simulink model "test2"  (R2016a)
settings: Solver=FixedStepAuto  SolverMode=SingleTasking  StartTime=0.0  StopTime=inf  FixedStep=5e-6  RelTol=1e-3
PreLoadFcn:
  | waijung.modelPreload; % Required for working with Waijung Blockset. Do not remove.
undefined symbols (not defined in the file): ARM, HSEOSC, Link, LQFP100, MDK, ST, STM32F407VE
libraries: simulink x8, powerlib_meascontrol x1, etargetslib x1, stm32f4_adc_lib x1, stm32f4_device_config_lib x1
CloseFcn:
  | waijung.modelClose; % Required for working with Waijung Blockset. Do not remove.
settings Model: Creator=Dang Khoa  LastModifiedBy=Dang Khoa
settings OptimizationCC: DefaultParameterBehavior=Inlined  OptimizeModelRefInitCode=on  LifeSpan=1
settings HardwareCC: ProdBitPerPointer=32  ProdLargestAtomicInteger=Long  ProdWordSize=32  ProdHWDeviceType=ARM Compatible->ARM 10  TargetEndianess=LittleEndian  TargetHWDeviceType=ARM Compatible->Cortex - M4
settings RTWCC: SystemTargetFile=stm32f4.tlc  GenCodeOnly=on  GenerateMakefile=off  TemplateMakefile=ert_default_tmf  Description=STM32F4 Target  GenerateReport=on  IncludeHyperlinkInReport=on  LaunchReport=on  GenerateTraceInfo=on  GenerateTraceReport=on  GenerateTraceReportSl=on  GenerateTraceReportSf=on  GenerateTraceReportEml=on
settings CodeAppCC: ForceParamTrailComments=on  IgnoreCustomStorageClasses=off  OperatorAnnotations=on  SimulinkDataObjDesc=on  SFDataObjDesc=on  MATLABFcnDesc=on  InsertBlockDesc=on  MATLABSourceComments=on
settings STFCustomTargetCC: ModelReferenceCompliant=off  CombineOutputUpdateFcns=on  ERTCustomFileBanners=on  SupportContinuousTime=off  SupportNonInlinedSFcns=off  MATLABClassNameForMDSCustomization=Simulink.SoftwareTarget.ERTCustomization  GRTInterface=off  SystemTargetFile=stm32f4.tlc
settings ERTTargetCC: ModelReferenceCompliant=off  ParMdlRefBuildCompliant=off  CompOptLevelCompliant=off  ConcurrentExecutionCompliant=off  ERTFirstTimeCompliant=off  ModelStepFunctionPrototypeControlCompliant=off  CPPClassGenCompliant=off  UseToolchainInfoCompliant=off  InlinedParameterPlacement=NonHierarchical  ERTSrcFileBannerTemplate=stm32f4_code_template.cgt  ERTHdrFileBannerTemplate=stm32f4_code_template.cgt  ERTDataSrcFileTemplate=stm32f4_code_template.cgt  ERTDataHdrFileTemplate=stm32f4_code_template.cgt  ERTCustomFileTemplate=stm32f4_file_process.tlc

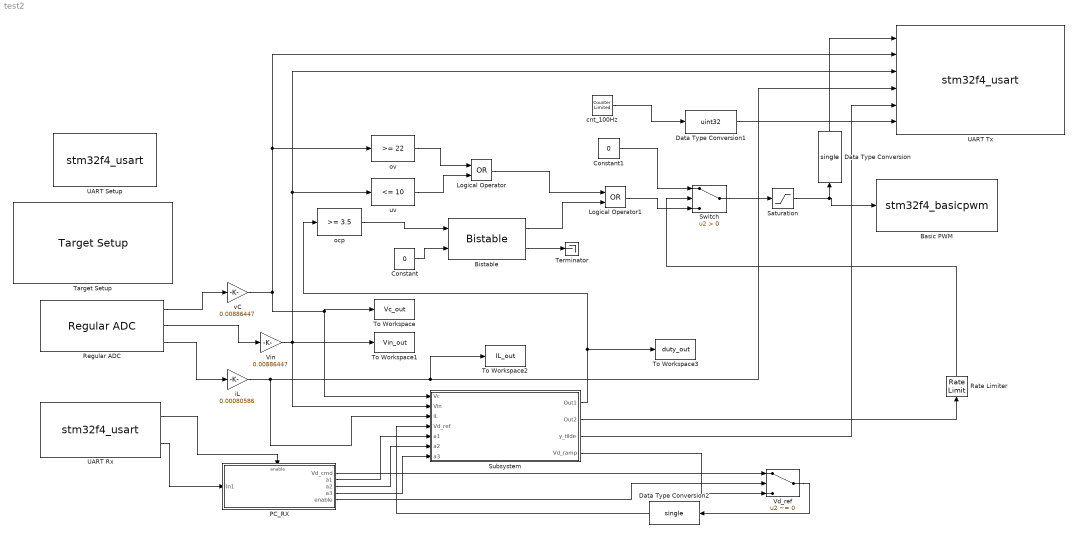
== system test2 ==
  Basic PWM : S-Function  FunctionName=stm32f4_basicpwm  Parameters=timer,pwmperiod,ch1pin,ch2pin,ch3pin,ch4pin,sampletime,sampletimestr,blockid,apb,portstr,pinstr,pinmat,timarr,timprescale,chmat,polaritystr  SFunctionDeploymentMode=off  EnableBusSupport=off  mask(stm32f4_basicpwm){timer=4, pwmperiod=1/20000, polarity=Active High, polaritystr=TIM_OCPolarity_High, ch1pin=B6, ch2pin=Not available - Do not use, ch3pin=Not available - Do not use, ch4pin=Not available - Do not use, sampletime=-1, sampletimestr=5e-05, blockid=BasicPWM, portpinstr=B6,,,, enablecustomportlabel=off, cinputportlabel=In1, In2, In3, In4, coutputportlabel=0, apb=1, portstr=["B"], pinstr=["GPIO_Pin_6"], pinmat=[1 6], timarr=64614, timprescale=25, chmat=[1]}
      mask prompts: pwmperiod "PWM Period (seconds)"; ch1pin "Channel 1"; ch2pin "Channel 2"; ch3pin "Channel 3"; ch4pin "Channel 4"; sampletime "Sample time (sec)"; sampletimestr "Compiled sample time (sec) in string"; portpinstr "Port pin string"; enablecustomportlabel "Enable custom port labels"; cinputportlabel "Custom input port labels (Ex. In1, In2, In3)"; coutputportlabel "Custom output port labels (Ex. Out1, Out2, Out3)"; portstr "Port string"; pinstr "Pin string"; pinmat "Pin matrix"; timarr "Timer ARR"; timprescale "Timer PRESCALE"; chmat "Channel order"
      mask help:
      | This block implements basic Edge-aligned Pulse Width Modulation (PWM) generation.
      | All timers are 16-bit. The PWM period is fixed (per timer).
      mask init:
      | stm32f4_basicpwm_callback('init');
      mask Help: web(fullfile(waijungdocroot,'stm32f4_basicpwm.htm'),'-browser')
      mask TypeOptions timer: 1 | 2 | 3 | 4 | 5 | 8 | 9 | 10 | 11 | 12 | 13 | 14
      mask Callback timer: stm32f4_basicpwm_callback('timer');
      mask Callback pwmperiod: stm32f4_basicpwm_callback('pwmperiod');
      mask TypeOptions polarity: Active High | Active Low
      mask Callback polarity: stm32f4_basicpwm_callback('polarity');
      mask TypeOptions ch1pin: Not available - Do not use | B6 | D12
      mask Callback ch1pin: stm32f4_basicpwm_callback('ch1pin');
      mask TypeOptions ch2pin: Not available - Do not use | B7 | D13
      mask Callback ch2pin: stm32f4_basicpwm_callback('ch2pin');
      mask TypeOptions ch3pin: Not available - Do not use | B8 | D14
      mask Callback ch3pin: stm32f4_basicpwm_callback('ch3pin');
      mask TypeOptions ch4pin: Not available - Do not use | B9 | D15
      mask Callback ch4pin: stm32f4_basicpwm_callback('ch4pin');
      mask Callback sampletime: stm32f4_basicpwm_callback('sampletime');
      mask Callback sampletimestr: stm32f4_basicpwm_callback('sampletimestr');
      mask Callback blockid: stm32f4_basicpwm_callback('blockid');
      mask Callback enablecustomportlabel: stm32f4_basicpwm_callback('enablecustomportlabel');
      mask Display: text(0.95, 0.5, 'Timer: 4\nPolarity: Active High\nPeriod (sec) 1/20000\nTs (sec): 5e-05','ver','middle','hor','right');port_label('input', 1,'CH1 (B6)')
  Bistable : powerlib_meascontrol/Logic/Bistable  Qpriority=Set  ic=0  Ts=-1
  Constant : Constant  Value=0
  Constant1 : Constant  Value=0
  Data Type Conversion : DataTypeConversion  OutDataTypeStr=single
  Data Type Conversion1 : DataTypeConversion  OutDataTypeStr=uint32
  Data Type Conversion2 : DataTypeConversion  OutDataTypeStr=single
  Logical Operator : Logic  Operator=OR  AllPortsSameDT=off  OutDataTypeStr=boolean
  Logical Operator1 : Logic  Operator=OR  AllPortsSameDT=off  OutDataTypeStr=boolean
  PC_RX : Subsystem  TreatAsAtomicUnit=on
  Rate Limiter : RateLimiter  RisingSlewLimit=2000  FallingSlewLimit=-4000  SampleTimeMode=inherited
  Regular ADC : stm32f4_adc_lib/Regular ADC  adcmodule=1  outputdatatype=Single  prescaler=2  prescalerstr=ADC_Prescaler_Div2  chsamplingtime=Auto  chsamplingtimestr=ADC_SampleTime_480Cycles  read_an0=off  read_an1=off  read_an2=off  read_an3=off  read_an4=off  read_an5=off  read_an6=off  read_an7=off  read_an8=off  read_an9=off  read_an10=on  read_an11=on  read_an12=on  read_an13=off  read_an14=off  read_an15=off  read_an16=off  read_an17=off  read_an18=off  pinstr=GPIO_Pin_10 | GPIO_Pin_11 | GPIO_Pin_12  usedpinarray="[0  0  0  0  0  0  0  0  0  0  1  1  1  0  0  0  0  0  0]"  usedportidarray="[2  2  2]"  usedpinidarray="[0  1  2]"  usedpinidcount=3  sampletime=5e-5  blockid=RegularADC  enablecustomportlabel=off  cinputportlabel=0  coutputportlabel=Out1, Out2
  Saturation : Saturate  UpperLimit=1  LowerLimit=0
  Subsystem : Subsystem
  Switch : Switch  Criteria=u2 > Threshold
  Target Setup : stm32f4_device_config_lib/Target Setup  Priority=100  compiler=MDK-ARM  previous_compiler=MDK-ARM  mcu=STM32F407VE (LQFP100)  mcustr=STM32F407VE  clockconfig=HSEOSC-8MHz  system_stm32f4xx_c_path=D:\MATLAB\setup\waijung17_03a\targets\stm32f4_target\stm32f4\utils\system_stm32f4xx_default\STM32F40_41xxx\hseosc8mhz  showmemoryconfiguration=off  stacksize=0x2000  heapsize=0x2000  enableautocompiledownload=on  fullchiperase=off  programmerinterface=ST-Link  editctrlstr=on  compilercontrolstr=-c --cpu Cortex-M4.fp -g -O3 --apcs=interwork --split_sections $(INCLUDES)  assemblercontrolstr="--cpu Cortex-M4.fp -g --apcs=interwork  --xref $(INCLUDES)"  linkercontrolstr="--cpu Cortex-M4.fp --strict --scatter \"$(MODELNAME).sct\" --summary_stderr --info summarysizes --map --xref --callgraph --symbols --info sizes --info totals --info unused --info veneers  --list \".\\$(MODELNAME).map\" -o $(MODELNAME).axf"  runafterdownload=on  execprofile=Real-time output  profileruart=3  profilerbaud=500000  profilertxpin=D8  profilerinitstr=5e-5,168000000,8400,500000,0  manualsetsampletime=on  sampletime=5e-5  blockid=TargetSetup  systickreloadvalue=8400  hseval=8000000  lastprofileruart=3  hclk=168000000  flashorigin=0x08000000  flashlength=0x80000  ramorigin=0x20000000  ramlength=0x20000  useextram=off
  Terminator : Terminator
  To Workspace : ToWorkspace  VariableName=Vc_out  SampleTime=-1
  To Workspace1 : ToWorkspace  VariableName=Vin_out  SampleTime=-1
  To Workspace2 : ToWorkspace  VariableName=IL_out  SampleTime=-1
  To Workspace3 : ToWorkspace  VariableName=duty_out  SampleTime=-1
  UART Rx : S-Function  Priority=1  FunctionName=stm32f4_usart  Parameters=configuration,uartmodule,transfer,baudrate,inputtype,outputtype,confstr,binheaderarray,binterminatorarray,asciiheader,asciiterminator,bindatalength,packetmode,varname,sampletime,sampletimestr,blockid  SFunctionDeploymentMode=off  EnableBusSupport=off  mask(stm32f4_usart){configuration=Rx, uartmodule=2, baudrate=115200, databits=8, parity=No, stopbit=1, remaptxpin=Not used, remaprxpin=Not used, flowcontrol=None, remapctspin=Not used, remaprtspin=Not used, advanceoptions=off, rxbuffersize=512, txbuffersize=512, transfer=Non-Blocking, packetmode=Binary Vector, binheader='00', binterminator='', porttype_double=0, porttype_single=0, porttype_int8=0, porttype_uint8=19, porttype_int16=0, porttype_uint16=0, porttype_int32=0, porttype_uint32=0, asciiformat='value=%d,%f', rx_asciiterminator=CRLF (0x0D 0x0A - "\r\n"), tx_asciiterminator=LF (0x0A - "\n"), storagename=<empty>, varname=, inputtype=[0], outputtype=[2 3  4867], binheaderarray=[1 0], binterminatorarray=[0 ], bindatalength=19, asciiheader='value=%d,%f\r\n', asciiterminator=[2 13 10], sampletime=5e-5, sampletimestr=5e-05, blockid=UARTRx, confstr=[ "dummy", "0", "*", "*", "0", "*", "*", "0", "*", "*", "0", "*", "*", "1", "4", "6", "1", "4", "5", "512", "512", "1", "2", "115200", "8", "No", "1", "None", "USART2"], lastmodule=1}
      mask prompts: uartmodule "UART Module"; baudrate "Baud rate (bps)"; databits "Data bits"; stopbit "Stop bit"; remaptxpin "Tx Pin"; remaprxpin "Rx Pin"; flowcontrol "Hardware flow control"; remapctspin "HW Flow control, CTS Pin"; remaprtspin "HW Flow control, RTS Pin"; advanceoptions "Advance options"; rxbuffersize "Rx buffer size (bytes)"; txbuffersize "Tx buffer size (bytes)"; packetmode "Packet mode"; binheader "Binary header (example: '7E 7E')"; binterminator "Binary terminator (example: '03 03')"; porttype_double "Number of data port, type DOUBLE"; porttype_single "Number of data port, type SINGLE"; porttype_int8 "Number of data port, type INT8"; porttype_uint8 "Number of data port, type UINT8"; porttype_int16 "Number of data port, type INT16"; porttype_uint16 "Number of data port, type UINT16"; porttype_int32 "Number of data port, type INT32"; porttype_uint32 "Number of data port, type UINT32"; asciiformat "Ascii format"; rx_asciiterminator "End of packet"; tx_asciiterminator "End of packet"; storagename "Buffer"; varname "Var name"; inputtype "Input data type"; outputtype "Output data type"; binheaderarray "Binary header"; binterminatorarray "Binary terminator"; bindatalength "Binary data length"; asciiheader "Ascii header (printf format)"; asciiterminator "Ascii terminator"; sampletime "Sample time (sec)"; sampletimestr "Compiled sample time (sec) in string"; confstr "Configuration string"; lastmodule "Last module selected"
      mask help:
      | Data type for Ascii format
      | %u, %i, %d, %o, %x: uint32
      | %e, %g, %f: single
      | %c: int8
      mask init:
      | stm32f4_usart_callback('init');
      mask Help: web(fullfile(waijungdocroot,'stm32f4_usart_rx.htm'), '-browser')
      mask TypeOptions configuration: Setup | Tx | Rx
      mask Callback configuration: stm32f4_usart_callback('configuration');
      mask TypeOptions uartmodule: 1 | 2 | 3 | 4 | 5 | 6
      mask Callback uartmodule: stm32f4_usart_callback('uartmodule');
      mask Callback baudrate: stm32f4_usart_callback('baudrate');
      mask TypeOptions databits: 8
      mask TypeOptions parity: No | Odd | Even
      mask TypeOptions stopbit: 0.5 | 1 | 1.5 | 2
      mask TypeOptions remaptxpin: Not used | A9 | B6
      mask TypeOptions remaprxpin: Not used | A10 | B7
      mask TypeOptions flowcontrol: None | RTS | CTS | RTS/CTS
      mask Callback flowcontrol: stm32f4_usart_callback('flowcontrol');
      mask TypeOptions remapctspin: Not used | A11
      mask TypeOptions remaprtspin: Not used | A12
      mask Callback advanceoptions: stm32f4_usart_callback('advanceoptions');
      mask TypeOptions rxbuffersize: 16 | 32 | 64 | 128 | 256 | 512 | 1024 | 2048
      mask TypeOptions txbuffersize: 16 | 32 | 64 | 128 | 256 | 512 | 1024 | 2048
      mask TypeOptions transfer: Blocking | Non-Blocking
      mask Callback transfer: stm32f4_usart_callback('transfer');
      mask TypeOptions packetmode: Ascii | Binary | Binary Vector | String Buffer | Raw Buffer | Read Line
      mask Callback packetmode: stm32f4_usart_callback('packetmode');
      mask Callback binheader: stm32f4_usart_callback('binheader');
      mask Callback binterminator: stm32f4_usart_callback('binterminator');
      mask Callback porttype_double: stm32f4_usart_callback('porttype');
      mask Callback porttype_single: stm32f4_usart_callback('porttype');
      mask Callback porttype_int8: stm32f4_usart_callback('porttype');
      mask Callback porttype_uint8: stm32f4_usart_callback('porttype');
      mask Callback porttype_int16: stm32f4_usart_callback('porttype');
      mask Callback porttype_uint16: stm32f4_usart_callback('porttype');
      mask Callback porttype_int32: stm32f4_usart_callback('porttype');
      mask Callback porttype_uint32: stm32f4_usart_callback('porttype');
      mask Callback asciiformat: stm32f4_usart_callback('asciiformat');
      mask TypeOptions rx_asciiterminator: CR (0x0D - "\r") | LF (0x0A - "\n") | CRLF (0x0D 0x0A - "\r\n")
      mask Callback rx_asciiterminator: stm32f4_usart_callback('rx_asciiterminator');
      mask TypeOptions tx_asciiterminator: CR (0x0D - "\r") | LF (0x0A - "\n") | CRLF (0x0D 0x0A - "\r\n") | None
      mask Callback tx_asciiterminator: stm32f4_usart_callback('tx_asciiterminator');
      mask TypeOptions storagename: <empty>
      mask Callback storagename: stm32f4_usart_callback('storagename');
      mask Callback varname: stm32f4_usart_callback('varname');
      mask Callback sampletime: stm32f4_usart_callback('sampletime');
      mask Callback sampletimestr: stm32f4_usart_callback('sampletimestr');
      mask Callback blockid: stm32f4_usart_callback('blockid');
      mask Display: text(0.05, 0.5, 'Module: USART2_Rx\nPacket: Binary Vector\nTransfer: Non-Blocking\nTs (sec): 5e-05','ver','middle','hor','left'); port_label('output', 1,'READY'); port_label('output', 2,'uint8(19)');
  UART Setup : S-Function  Priority=1  FunctionName=stm32f4_usart  Parameters=configuration,uartmodule,transfer,baudrate,inputtype,outputtype,confstr,binheaderarray,binterminatorarray,asciiheader,asciiterminator,bindatalength,packetmode,varname,sampletime,sampletimestr,blockid  SFunctionDeploymentMode=off  EnableBusSupport=off  mask(stm32f4_usart){configuration=Setup, uartmodule=2, baudrate=115200, databits=8, parity=No, stopbit=1, remaptxpin=A2, remaprxpin=A3, flowcontrol=None, remapctspin=Not used, remaprtspin=Not used, advanceoptions=off, rxbuffersize=512, txbuffersize=512, transfer=Blocking, packetmode=Ascii, binheader='7E 7E', binterminator='03 03', porttype_double=1, porttype_single=0, porttype_int8=1, porttype_uint8=0, porttype_int16=0, porttype_uint16=0, porttype_int32=0, porttype_uint32=0, asciiformat='%d,%f', rx_asciiterminator=CRLF (0x0D 0x0A - "\r\n"), tx_asciiterminator=CR (0x0D - "\r"), storagename=<empty>, varname=, inputtype=[0], outputtype=[0], binheaderarray=[0], binterminatorarray=[0], bindatalength=0, asciiheader='', asciiterminator=[0], sampletime=-1, sampletimestr=5e-05, blockid=UARTSetup, confstr=[ "dummy", "1", "A", "2", "1", "A", "3", "0", "*", "*", "0", "*", "*", "1", "4", "6", "1", "4", "5", "512", "512", "1", "2", "115200", "8", "No", "1", "None", "USART2"], lastmodule=2}
      mask prompts: uartmodule "UART Module"; baudrate "Baud rate (bps)"; databits "Data bits"; stopbit "Stop bit"; remaptxpin "Tx Pin"; remaprxpin "Rx Pin"; flowcontrol "Hardware flow control"; remapctspin "HW Flow control, CTS Pin"; remaprtspin "HW Flow control, RTS Pin"; advanceoptions "Advance options"; rxbuffersize "Rx buffer size (bytes)"; txbuffersize "Tx buffer size (bytes)"; packetmode "Packet mode"; binheader "Binary header (example: '7E 7E')"; binterminator "Binary terminator (example: '03 03')"; porttype_double "Number of data port, type DOUBLE"; porttype_single "Number of data port, type SINGLE"; porttype_int8 "Number of data port, type INT8"; porttype_uint8 "Number of data port, type UINT8"; porttype_int16 "Number of data port, type INT16"; porttype_uint16 "Number of data port, type UINT16"; porttype_int32 "Number of data port, type INT32"; porttype_uint32 "Number of data port, type UINT32"; asciiformat "Ascii format"; rx_asciiterminator "End of packet"; tx_asciiterminator "End of packet"; storagename "Buffer"; varname "Var name"; inputtype "Input data type"; outputtype "Output data type"; binheaderarray "Binary header"; binterminatorarray "Binary terminator"; bindatalength "Binary data length"; asciiheader "Ascii header (printf format)"; asciiterminator "Ascii terminator"; sampletime "Sample time (sec)"; sampletimestr "Compiled sample time (sec) in string"; confstr "Configuration string"; lastmodule "Last module selected"
      mask help:
      | Default STM32F4DISCOVERY + aMG F4 Connect 2 + aMG USB Converter N2 settings use
      |
      | USART3, Tx D8, Rx D9 and USB Serial Converter A.
      mask init:
      | stm32f4_usart_callback('init');
      mask Help: web(fullfile(waijungdocroot,'stm32f4_usart_setup.htm'), '-browser')
      mask TypeOptions configuration: Setup | Tx | Rx
      mask Callback configuration: stm32f4_usart_callback('configuration');
      mask TypeOptions uartmodule: 1 | 2 | 3 | 4 | 5 | 6
      mask Callback uartmodule: stm32f4_usart_callback('uartmodule');
      mask Callback baudrate: stm32f4_usart_callback('baudrate');
      mask TypeOptions databits: 8
      mask TypeOptions parity: No | Odd | Even
      mask TypeOptions stopbit: 0.5 | 1 | 1.5 | 2
      mask TypeOptions remaptxpin: Not used | A2 | D5
      mask TypeOptions remaprxpin: Not used | A3 | D6
      mask TypeOptions flowcontrol: None | RTS | CTS | RTS/CTS
      mask Callback flowcontrol: stm32f4_usart_callback('flowcontrol');
      mask TypeOptions remapctspin: Not used | A0 | D3
      mask TypeOptions remaprtspin: Not used | A1 | D4
      mask Callback advanceoptions: stm32f4_usart_callback('advanceoptions');
      mask TypeOptions rxbuffersize: 16 | 32 | 64 | 128 | 256 | 512 | 1024 | 2048
      mask TypeOptions txbuffersize: 16 | 32 | 64 | 128 | 256 | 512 | 1024 | 2048
      mask TypeOptions transfer: Blocking | Non-Blocking
      mask Callback transfer: stm32f4_usart_callback('transfer');
      mask TypeOptions packetmode: Ascii | Binary | String Buffer
      mask Callback packetmode: stm32f4_usart_callback('packetmode');
      mask Callback binheader: stm32f4_usart_callback('binheader');
      mask Callback binterminator: stm32f4_usart_callback('binterminator');
      mask Callback porttype_double: stm32f4_usart_callback('porttype');
      mask Callback porttype_single: stm32f4_usart_callback('porttype');
      mask Callback porttype_int8: stm32f4_usart_callback('porttype');
      mask Callback porttype_uint8: stm32f4_usart_callback('porttype');
      mask Callback porttype_int16: stm32f4_usart_callback('porttype');
      mask Callback porttype_uint16: stm32f4_usart_callback('porttype');
      mask Callback porttype_int32: stm32f4_usart_callback('porttype');
      mask Callback porttype_uint32: stm32f4_usart_callback('porttype');
      mask Callback asciiformat: stm32f4_usart_callback('asciiformat');
      mask TypeOptions rx_asciiterminator: CR (0x0D - "\r") | LF (0x0A - "\n") | CRLF (0x0D 0x0A - "\r\n")
      mask Callback rx_asciiterminator: stm32f4_usart_callback('rx_asciiterminator');
      mask TypeOptions tx_asciiterminator: CR (0x0D - "\r") | LF (0x0A - "\n") | CRLF (0x0D 0x0A - "\r\n") | None
      mask Callback tx_asciiterminator: stm32f4_usart_callback('tx_asciiterminator');
      mask TypeOptions storagename: <empty>
      mask Callback storagename: stm32f4_usart_callback('storagename');
      mask Callback varname: stm32f4_usart_callback('varname');
      mask Callback sampletime: stm32f4_usart_callback('sampletime');
      mask Callback sampletimestr: stm32f4_usart_callback('sampletimestr');
      mask Callback blockid: stm32f4_usart_callback('blockid');
      mask Display: text(0.5, 0.5, 'Module: USART2_Setup\nBaud (Bps): 115200\nDMA Buffer: 512/512\nTx/Rx Pin: A2/A3','ver','middle','hor','center');
  UART Tx : S-Function  Priority=1  FunctionName=stm32f4_usart  Parameters=configuration,uartmodule,transfer,baudrate,inputtype,outputtype,confstr,binheaderarray,binterminatorarray,asciiheader,asciiterminator,bindatalength,packetmode,varname,sampletime,sampletimestr,blockid  SFunctionDeploymentMode=off  EnableBusSupport=off  mask(stm32f4_usart){configuration=Tx, uartmodule=2, baudrate=115200, databits=8, parity=No, stopbit=1, remaptxpin=Not used, remaprxpin=Not used, flowcontrol=None, remapctspin=Not used, remaprtspin=Not used, advanceoptions=off, rxbuffersize=512, txbuffersize=512, transfer=Non-Blocking, packetmode=Binary, binheader='AA 55', binterminator='', porttype_double=0, porttype_single=5, porttype_int8=0, porttype_uint8=0, porttype_int16=0, porttype_uint16=0, porttype_int32=0, porttype_uint32=1, asciiformat='value=%d,%f', rx_asciiterminator=CRLF (0x0D 0x0A - "\r\n"), tx_asciiterminator=CRLF (0x0D 0x0A - "\r\n"), storagename=<empty>, varname=, inputtype=[6  1 1 1 1 1 7], outputtype=[0], binheaderarray=[2 170   85], binterminatorarray=[0 ], bindatalength=24, asciiheader='value=%d,%f\r\n', asciiterminator=[2 13 10], sampletime=-1, sampletimestr=5e-05, blockid=UARTTx, confstr=[ "dummy", "0", "*", "*", "0", "*", "*", "0", "*", "*", "0", "*", "*", "1", "4", "6", "1", "4", "5", "512", "512", "1", "2", "115200", "8", "No", "1", "None", "USART2"], lastmodule=1}
      mask prompts: uartmodule "UART Module"; baudrate "Baud rate (bps)"; databits "Data bits"; stopbit "Stop bit"; remaptxpin "Tx Pin"; remaprxpin "Rx Pin"; flowcontrol "Hardware flow control"; remapctspin "HW Flow control, CTS Pin"; remaprtspin "HW Flow control, RTS Pin"; advanceoptions "Advance options"; rxbuffersize "Rx buffer size (bytes)"; txbuffersize "Tx buffer size (bytes)"; packetmode "Packet mode"; binheader "Binary header (example: '7E 7E')"; binterminator "Binary terminator (example: '03 03')"; porttype_double "Number of data port, type DOUBLE"; porttype_single "Number of data port, type SINGLE"; porttype_int8 "Number of data port, type INT8"; porttype_uint8 "Number of data port, type UINT8"; porttype_int16 "Number of data port, type INT16"; porttype_uint16 "Number of data port, type UINT16"; porttype_int32 "Number of data port, type INT32"; porttype_uint32 "Number of data port, type UINT32"; asciiformat "Ascii format"; rx_asciiterminator "End of packet"; tx_asciiterminator "End of packet"; storagename "Buffer"; varname "Var name"; inputtype "Input data type"; outputtype "Output data type"; binheaderarray "Binary header"; binterminatorarray "Binary terminator"; bindatalength "Binary data length"; asciiheader "Ascii header (printf format)"; asciiterminator "Ascii terminator"; sampletime "Sample time (sec)"; sampletimestr "Compiled sample time (sec) in string"; confstr "Configuration string"; lastmodule "Last module selected"
      mask help:
      | Data type for Ascii format
      | %u, %i, %d, %o, %x: uint32
      | %e, %g, %f: single
      | %c: int8
      mask init:
      | stm32f4_usart_callback('init');
      mask Help: web(fullfile(waijungdocroot,'stm32f4_usart_tx.htm'), '-browser')
      mask TypeOptions configuration: Setup | Tx | Rx
      mask Callback configuration: stm32f4_usart_callback('configuration');
      mask TypeOptions uartmodule: 1 | 2 | 3 | 4 | 5 | 6
      mask Callback uartmodule: stm32f4_usart_callback('uartmodule');
      mask Callback baudrate: stm32f4_usart_callback('baudrate');
      mask TypeOptions databits: 8
      mask TypeOptions parity: No | Odd | Even
      mask TypeOptions stopbit: 0.5 | 1 | 1.5 | 2
      mask TypeOptions remaptxpin: Not used | A9 | B6
      mask TypeOptions remaprxpin: Not used | A10 | B7
      mask TypeOptions flowcontrol: None | RTS | CTS | RTS/CTS
      mask Callback flowcontrol: stm32f4_usart_callback('flowcontrol');
      mask TypeOptions remapctspin: Not used | A11
      mask TypeOptions remaprtspin: Not used | A12
      mask Callback advanceoptions: stm32f4_usart_callback('advanceoptions');
      mask TypeOptions rxbuffersize: 16 | 32 | 64 | 128 | 256 | 512 | 1024 | 2048
      mask TypeOptions txbuffersize: 16 | 32 | 64 | 128 | 256 | 512 | 1024 | 2048
      mask TypeOptions transfer: Blocking | Non-Blocking
      mask Callback transfer: stm32f4_usart_callback('transfer');
      mask TypeOptions packetmode: Ascii | Binary | Binary Vector | String Buffer | Raw Buffer
      mask Callback packetmode: stm32f4_usart_callback('packetmode');
      mask Callback binheader: stm32f4_usart_callback('binheader');
      mask Callback binterminator: stm32f4_usart_callback('binterminator');
      mask Callback porttype_double: stm32f4_usart_callback('porttype');
      mask Callback porttype_single: stm32f4_usart_callback('porttype');
      mask Callback porttype_int8: stm32f4_usart_callback('porttype');
      mask Callback porttype_uint8: stm32f4_usart_callback('porttype');
      mask Callback porttype_int16: stm32f4_usart_callback('porttype');
      mask Callback porttype_uint16: stm32f4_usart_callback('porttype');
      mask Callback porttype_int32: stm32f4_usart_callback('porttype');
      mask Callback porttype_uint32: stm32f4_usart_callback('porttype');
      mask Callback asciiformat: stm32f4_usart_callback('asciiformat');
      mask TypeOptions rx_asciiterminator: CR (0x0D - "\r") | LF (0x0A - "\n") | CRLF (0x0D 0x0A - "\r\n")
      mask Callback rx_asciiterminator: stm32f4_usart_callback('rx_asciiterminator');
      mask TypeOptions tx_asciiterminator: CR (0x0D - "\r") | LF (0x0A - "\n") | CRLF (0x0D 0x0A - "\r\n") | None
      mask Callback tx_asciiterminator: stm32f4_usart_callback('tx_asciiterminator');
      mask TypeOptions storagename: <empty>
      mask Callback storagename: stm32f4_usart_callback('storagename');
      mask Callback varname: stm32f4_usart_callback('varname');
      mask Callback sampletime: stm32f4_usart_callback('sampletime');
      mask Callback sampletimestr: stm32f4_usart_callback('sampletimestr');
      mask Callback blockid: stm32f4_usart_callback('blockid');
      mask Display: text(0.5, 0.5, 'Module: USART2_Tx\nPacket: Binary\nTransfer: Non-Blocking\nTs (sec): 5e-05','ver','middle','hor','center'); port_label('input', 1,'single'); port_label('input', 2,'single'); port_label('input', 3,'single'); port_label('input', 4,'single'); port_label('input', 5,'single'); port_label('input', 6,'uint32');
  Vd_ref : Switch  Criteria=u2 ~= 0
  Vin : Gain  Gain=0.00886447
  cnt_100Hz : simulink/Sources/Counter Limited  uplimit=199  tsamp=5e-5
  iL : Gain  Gain=0.00080586
  ocp : simulink/Logic and Bit Operations/Compare To Constant  relop=>=  const=3.5  OutDataTypeStr=boolean
  ov : simulink/Logic and Bit Operations/Compare To Constant  relop=>=  const=22  OutDataTypeStr=boolean
  uv : simulink/Logic and Bit Operations/Compare To Constant  relop=<=  const=10  OutDataTypeStr=boolean
  vC : Gain  Gain=0.00886447
  wires:
  Regular ADC/2 -> Vin/1
  Regular ADC/1 -> vC/1
  vC/1 -> UART Tx/2, ov/1, Subsystem/1(Vc), To Workspace/1
  Vin/1 -> To Workspace1/1, UART Tx/3, uv/1, Subsystem/2(Vin)
  uv/1 -> Logical Operator/2
  ov/1 -> Logical Operator/1
  ocp/1 -> Bistable/1
  Constant/1 -> Bistable/2
  Logical Operator/1 -> Logical Operator1/1
  Bistable/1 -> Logical Operator1/2
  Constant1/1 -> Switch/1
  Logical Operator1/1 -> Switch/3
  Rate Limiter/1 -> Switch/2
  Switch/1 -> Saturation/1
  Saturation/1 -> Basic PWM/1, Data Type Conversion/1
  Subsystem/1(Out1) -> To Workspace3/1, ocp/1
  Subsystem/2(Out2) -> Rate Limiter/1
  iL/1 -> To Workspace2/1, UART Tx/4, Subsystem/3("iL ")
  Regular ADC/3 -> iL/1
  Subsystem/3(y_tilde) -> UART Tx/5
  UART Rx/1 -> PC_RX/Enable
  PC_RX/1(Vd_cmd) -> Vd_ref/1
  PC_RX/5(enable) -> Vd_ref/2
  Subsystem/4(Vd_ramp) -> Vd_ref/3
  PC_RX/2(a1) -> Subsystem/5(a1)
  PC_RX/3(a2) -> Subsystem/6(a2)
  PC_RX/4(a3) -> Subsystem/7(a3)
  Bistable/2 -> Terminator/1
  UART Rx/2 -> PC_RX/1(In1)
  Data Type Conversion/1 -> UART Tx/1
  Data Type Conversion1/1 -> UART Tx/6
  cnt_100Hz/1 -> Data Type Conversion1/1
  Vd_ref/1 -> Data Type Conversion2/1
  Data Type Conversion2/1 -> Subsystem/4(Vd_ref)

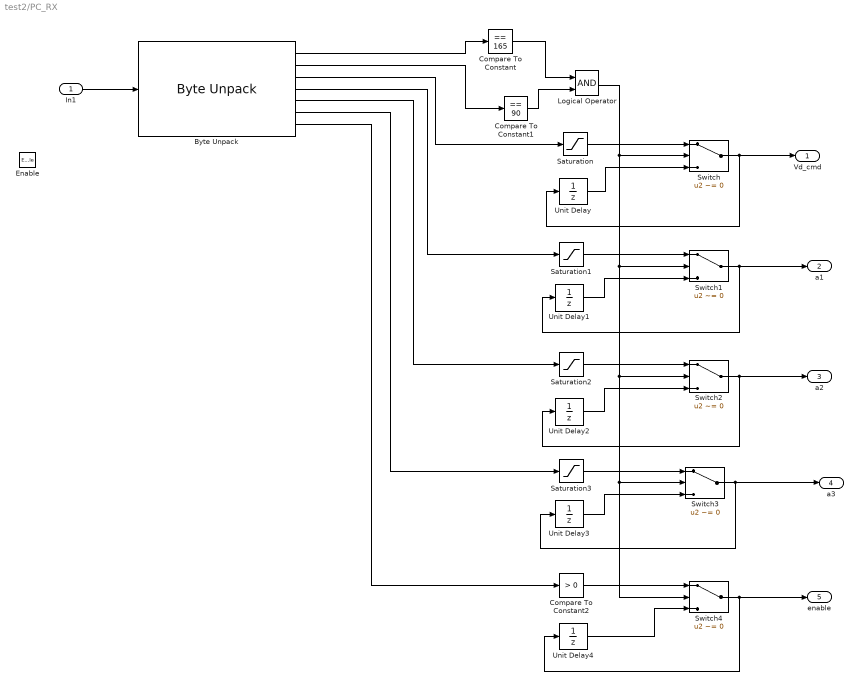
== system test2/PC_RX ==
  In1 : Inport  OutDataTypeStr=uint8  PortDimensions=19
  Enable : EnablePort
  Byte Unpack : etargetslib/Byte Unpack  dimensions={[1],[1],[1],[1],[1],[1],[1]}  datatypes={'uint8','uint8','single','single','single','single','uint8'}  byteAlign=1
  Compare To Constant : simulink/Logic and Bit Operations/Compare To Constant  relop===  const=165  OutDataTypeStr=boolean
  Compare To Constant1 : simulink/Logic and Bit Operations/Compare To Constant  relop===  const=90  OutDataTypeStr=boolean
  Compare To Constant2 : simulink/Logic and Bit Operations/Compare To Constant  relop=>  const=0  OutDataTypeStr=boolean
  Logical Operator : Logic  AllPortsSameDT=off  OutDataTypeStr=boolean
  Saturation : Saturate  UpperLimit=25  LowerLimit=15
  Saturation1 : Saturate  UpperLimit=1  LowerLimit=0
  Saturation2 : Saturate  UpperLimit=0.2  LowerLimit=0
  Saturation3 : Saturate  UpperLimit=0.1  LowerLimit=0
  Switch{,1..4} (5 alike) : Switch  Criteria=u2 ~= 0
  Unit Delay : UnitDelay  InitialCondition=20  SampleTime=-1
  Unit Delay1 : UnitDelay  InitialCondition=0.2  SampleTime=-1
  Unit Delay2 : UnitDelay  SampleTime=-1
  Unit Delay3 : UnitDelay  SampleTime=-1
  Unit Delay4 : UnitDelay  SampleTime=-1
  Vd_cmd : Outport  OutDataTypeStr=single
  a1 : Outport  Port=2  OutDataTypeStr=single
  a2 : Outport  Port=3  OutDataTypeStr=single
  a3 : Outport  Port=4  OutDataTypeStr=single
  enable : Outport  Port=5  OutDataTypeStr=boolean
  wires:
  In1/1 -> Byte Unpack/1
  Compare To Constant/1 -> Logical Operator/1
  Compare To Constant1/1 -> Logical Operator/2
  Byte Unpack/1 -> Compare To Constant/1
  Byte Unpack/2 -> Compare To Constant1/1
  Byte Unpack/3 -> Saturation/1
  Byte Unpack/4 -> Saturation1/1
  Byte Unpack/5 -> Saturation2/1
  Byte Unpack/6 -> Saturation3/1
  Byte Unpack/7 -> Compare To Constant2/1
  Logical Operator/1 -> Switch4/2, Switch3/2, Switch2/2, Switch1/2, Switch/2
  Saturation/1 -> Switch/1
  Saturation1/1 -> Switch1/1
  Saturation2/1 -> Switch2/1
  Saturation3/1 -> Switch3/1
  Compare To Constant2/1 -> Switch4/1
  Unit Delay/1 -> Switch/3
  Switch/1 -> Vd_cmd/1, Unit Delay/1
  Unit Delay1/1 -> Switch1/3
  Switch1/1 -> a1/1, Unit Delay1/1
  Unit Delay2/1 -> Switch2/3
  Switch2/1 -> a2/1, Unit Delay2/1
  Unit Delay3/1 -> Switch3/3
  Switch3/1 -> Unit Delay3/1, a3/1
  Unit Delay4/1 -> Switch4/3
  Switch4/1 -> enable/1, Unit Delay4/1

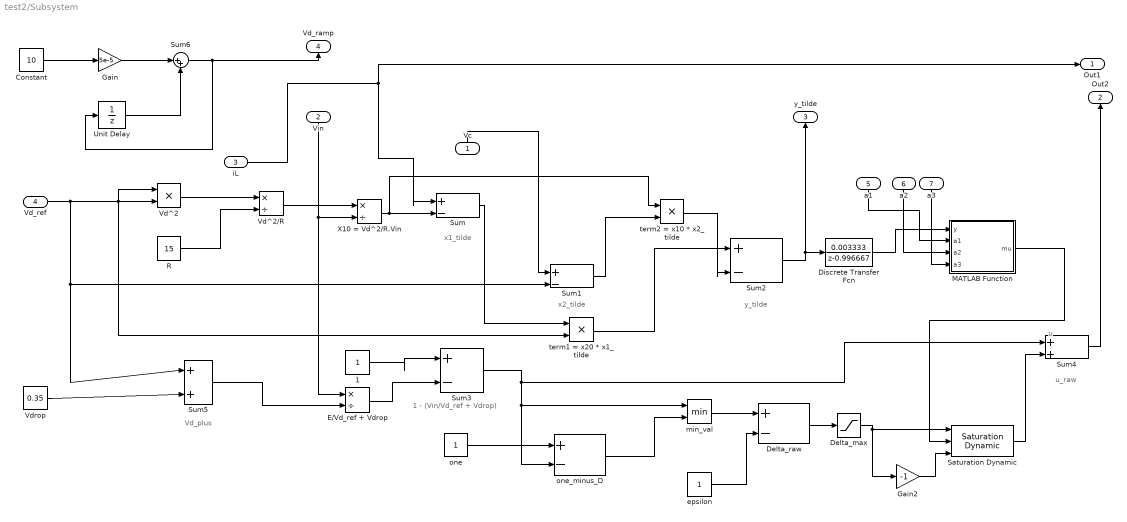
== system test2/Subsystem ==
  note: Vd_plus
  note: u_raw
  note: u
  note: 1 - (Vin/Vd_ref + Vdrop)
  note: x1_tilde
  note: x2_tilde
  note: y_tilde
  Vc : Inport
  Vin : Inport  Port=2
  "iL " : Inport  Port=3
  Vd_ref : Inport  Port=4
  a1 : Inport  Port=5
  a2 : Inport  Port=6
  a3 : Inport  Port=7
  "1 " : Constant
  Constant : Constant  Value=10
  Delta_max : Saturate  UpperLimit=inf  LowerLimit=0
  Delta_raw : Sum  Inputs=+-
  Discrete Transfer Fcn : DiscreteTransferFcn  Numerator=[0.003333]  Denominator=[1 -0.996667]  SampleTime=5e-5
  E/Vd_ref + Vdrop : Product  Inputs=*/
  Gain : Gain  Gain=5e-5
  Gain2 : Gain  Gain=-1  OutDataTypeStr=single
  MATLAB Function : MATLAB Function  TreatAsAtomicUnit=on
  R : Constant  Value=15  OutDataTypeStr=single
  Saturation Dynamic : simulink/Discontinuities/Saturation Dynamic  OutMin=[]  OutMax=[]  OutDataTypeStr=Inherit: Same as second input  OutDataType=fixdt(1, 16)  OutScaling=2^-10  DoSatur=off
  Sum : Sum  Inputs=|+-
  Sum1 : Sum  Inputs=|+-  OutDataTypeStr=Inherit: Same as first input
  Sum2 : Sum  Inputs=|+-
  Sum3 : Sum  Inputs=|+-
  Sum4 : Sum  Inputs=|++
  Sum5 : Sum  Inputs=|++
  Sum6 : Sum  Inputs=|++
  Unit Delay : UnitDelay  SampleTime=5e-5
  Vd^2 : Product  OutDataTypeStr=Inherit: Same as first input
  Vd^2/R : Product  Inputs=*/
  Vdrop : Constant  Value=0.35  OutDataTypeStr=single
  X10 = Vd^2/R.Vin : Product  Inputs=*/  OutDataTypeStr=Inherit: Same as first input
  epsilon : Constant  OutDataTypeStr=single
  min_val : MinMax  Inputs=2
  one : Constant  OutDataTypeStr=single
  one_minus_D : Sum  Inputs=+-
  term1 = x20 * x1_tilde : Product  OutDataTypeStr=Inherit: Same as first input
  term2 = x10 * x2_tilde : Product  OutDataTypeStr=Inherit: Same as first input
  Out1 : Outport
  Out2 : Outport  Port=2
  y_tilde : Outport  Port=3
  Vd_ramp : Outport  Port=4
  wires:
  "1 "/1 -> Sum3/1
  one_minus_D/1 -> min_val/2
  Vd^2/1 -> Vd^2/R/1
  R/1 -> Vd^2/R/2
  Delta_raw/1 -> Delta_max/1
  Delta_max/1 -> Gain2/1, Saturation Dynamic/1
  Vd^2/R/1 -> X10 = Vd^2/R.Vin/1
  one/1 -> one_minus_D/1
  term2 = x10 * x2_tilde/1 -> Sum2/2
  Gain2/1 -> Saturation Dynamic/3
  X10 = Vd^2/R.Vin/1 -> Sum/2, term2 = x10 * x2_tilde/1
  term1 = x20 * x1_tilde/1 -> Sum2/1
  Sum3/1 -> Sum4/1, one_minus_D/2, min_val/1
  min_val/1 -> Delta_raw/1
  epsilon/1 -> Delta_raw/2
  Vd_ref/1 -> term1 = x20 * x1_tilde/2, Vd^2/1, Vd^2/2, Sum1/2, Sum5/1
  Sum1/1 -> term2 = x10 * x2_tilde/2
  Sum/1 -> term1 = x20 * x1_tilde/1
  E/Vd_ref + Vdrop/1 -> Sum3/2
  Discrete Transfer Fcn/1 -> MATLAB Function/1(y)
  Saturation Dynamic/1 -> Sum4/2
  Vdrop/1 -> Sum5/2
  MATLAB Function/1(mu) -> Saturation Dynamic/2
  Sum5/1 -> E/Vd_ref + Vdrop/2
  "iL "/1 -> Sum/1, Out1/1
  Sum4/1 -> Out2/1
  Vin/1 -> X10 = Vd^2/R.Vin/2, E/Vd_ref + Vdrop/1
  Sum2/1 -> y_tilde/1, Discrete Transfer Fcn/1
  Vc/1 -> Sum1/1
  a1/1 -> MATLAB Function/2(a1)
  a2/1 -> MATLAB Function/3(a2)
  a3/1 -> MATLAB Function/4(a3)
  Sum6/1 -> Unit Delay/1, Vd_ramp/1
  Constant/1 -> Gain/1
  Gain/1 -> Sum6/1
  Unit Delay/1 -> Sum6/2

== matlab function test2/Subsystem/MATLAB Function ==
  data: y input; mu output; a1 input; a2 input; a3 input
function mu = PBCphi(y, a1, a2, a3)
%#codegen
% y,a1,a2,a3 đều single
mu = -(a1*y + a2*y*y*y + a3*y*y*y*y*y);
end
